simulink model "Planta_con_gravedad"  (R2020a)
settings: Solver=VariableStepAuto  StartTime=0.0  StopTime=10.0  RelTol=1e-3
undefined symbols (not defined in the file): bm, g, K_motor, L, m_total, R
settings Model: Creator=Adriana  LastModifiedBy=Adriana

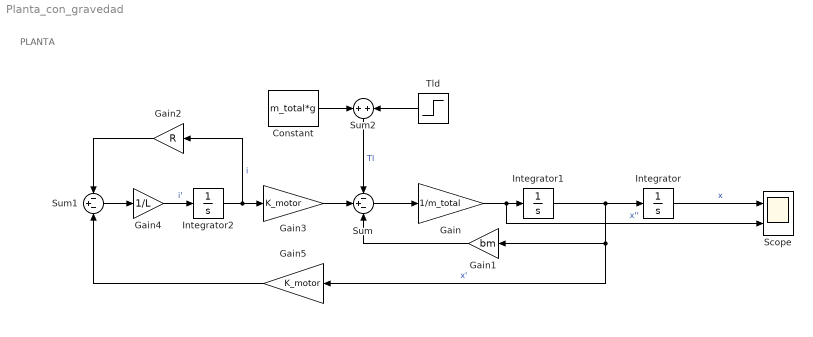
== system Planta_con_gravedad ==
  note: PLANTA
  Constant : Constant  Value=m_total*g
  Gain : Gain  Gain=1/m_total
  Gain1 : Gain  Gain=bm
  Gain2 : Gain  Gain=R
  Gain3 : Gain  Gain=K_motor
  Gain4 : Gain  Gain=1/L
  Gain5 : Gain  Gain=K_motor
  Integrator : Integrator
  Integrator1 : Integrator
  Integrator2 : Integrator
  Scope : Scope  NumInputPorts=2
  Sum : Sum  Inputs=-+-
  Sum1 : Sum  Inputs=-+-
  Sum2 : Sum
  Tld : Step  SampleTime=0
  wires:
  Integrator1/1 -> Gain5/1, Gain1/1, Integrator/1  "x'"
  Integrator/1 -> Scope/1  "x"
  Gain/1 -> Scope/2, Integrator1/1  "x''"
  Sum/1 -> Gain/1
  Gain1/1 -> Sum/3
  Sum2/1 -> Sum/1  "Tl"
  Gain3/1 -> Sum/2
  Integrator2/1 -> Gain2/1, Gain3/1  "i"
  Sum1/1 -> Gain4/1
  Gain4/1 -> Integrator2/1  "i'"
  Gain2/1 -> Sum1/1
  Gain5/1 -> Sum1/3
  ? -> Sum1/2  "V*"
  Constant/1 -> Sum2/1
  Tld/1 -> Sum2/2
